simulink model "example_rotor_response"  (R2016a)
settings: Solver=VariableStepAuto  StartTime=0.0  StopTime=15  RelTol=1e-3
settings Model: Creator=mgreiff  LastModifiedBy=mgreiff

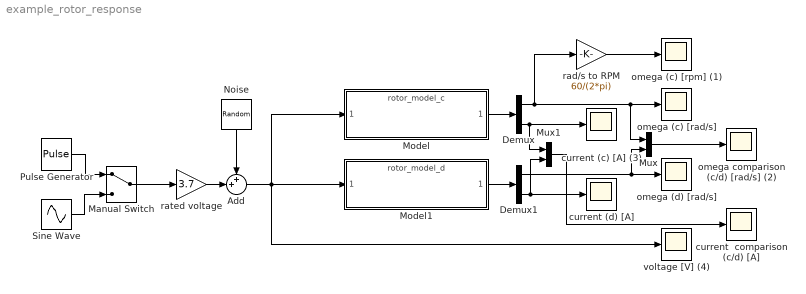
== system example_rotor_response ==
  Add : Sum  Inputs=++|
  Demux : Demux  Outputs=2
  Demux1 : Demux  Outputs=2
  Manual Switch : ManualSwitch
  Model : ModelReference  ModelNameDialog=rotor_model_c.slx  SimulationMode=Normal  ModelReferenceVersion=1.28
  Model1 : ModelReference  ModelNameDialog=rotor_model_d.slx  SimulationMode=Normal  ModelReferenceVersion=1.28
  Mux : Mux  Inputs=2
  Mux1 : Mux  Inputs=2
  Noise : RandomNumber  Variance=0.001  SampleTime=0.002
  Pulse Generator : DiscretePulseGenerator  PulseType=Time based  Period=4  PulseWidth=50  PhaseDelay=0.6
  Sine Wave : Sin  SampleTime=0
  current  comparison (c/d) [A] : Scope
  current (c) [A] (3) : Scope
  current (d) [A] : Scope
  omega (c) [rad/s] : Scope
  omega (c) [rpm] (1) : Scope
  omega (d) [rad/s] : Scope
  omega comparison (c/d) [rad/s] (2) : Scope
  rad/s to RPM : Gain  Gain=60/(2*pi)
  rated voltage : Gain  Gain=3.7
  voltage [V] (4) : Scope
  wires:
  Add/1 -> Model/1, voltage [V] (4)/1, Model1/1
  Noise/1 -> Add/1
  Sine Wave/1 -> Manual Switch/2
  Pulse Generator/1 -> Manual Switch/1
  Manual Switch/1 -> rated voltage/1
  rated voltage/1 -> Add/2
  Model/1 -> Demux/1
  Demux/1 -> rad/s to RPM/1, omega (c) [rad/s]/1, Mux/1
  Demux/2 -> Mux1/1, current (c) [A] (3)/1
  rad/s to RPM/1 -> omega (c) [rpm] (1)/1
  Model1/1 -> Demux1/1
  Demux1/1 -> Mux/2, omega (d) [rad/s]/1
  Demux1/2 -> current (d) [A]/1, Mux1/2
  Mux/1 -> omega comparison (c/d) [rad/s] (2)/1
  Mux1/1 -> current  comparison (c/d) [A]/1
